simulink model "problem8"  (R2020b)
settings: Solver=VariableStepAuto  StartTime=0.0  StopTime=20  RelTol=1e-3
libraries: simulink x1
settings Model: EnablePacing=on  Creator=INDRAJIT MARATHE  LastModifiedBy=Acer

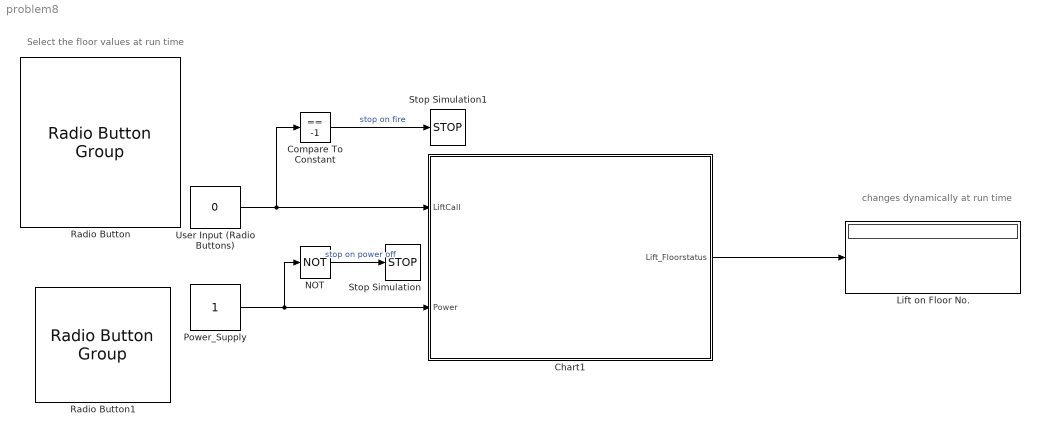
== system problem8 ==
  note: changes dynamically at run time
  note: Select the floor values at run time
  Chart1 : Stateflow chart  TreatAsAtomicUnit=on
  Compare To Constant : simulink/Logic and Bit Operations/Compare To Constant  relop===  const=-1  OutDataTypeStr=boolean
  Lift on Floor No. : Display
  NOT : Logic  Operator=NOT  IconShape=distinctive  AllPortsSameDT=off  OutDataTypeStr=boolean
  Power_Supply : Constant
  Radio Button : RadioButtonGroup  SelectedLabel=Ground Floor  ButtonGroupName=Lift Dashboard
      settings: Values={{'1', '2', '3', '4', '5', 'Ground Floor', 'Fire'}, [1 2 3 4 5 0 -1]}
  Radio Button1 : RadioButtonGroup  SelectedLabel=On  ButtonGroupName=Power Supply
      settings: Values={{'On', 'Off'}, [1 0]}
  Stop Simulation : Stop
  Stop Simulation1 : Stop
  User Input (Radio Buttons) : Constant  Value=0
  wires:
  Power_Supply/1 -> NOT/1, Chart1/2(Power)
  Chart1/1(Lift_Floorstatus) -> Lift on Floor No./1
  User Input (Radio Buttons)/1 -> Compare To Constant/1, Chart1/1(LiftCall)
  NOT/1 -> Stop Simulation/1  "stop on power off"
  Compare To Constant/1 -> Stop Simulation1/1  "stop on fire"

== stateflow chart problem8/Chart1 ==
  state PowerControl [parallel]
    settings: executionOrder=1
    state Idle
      Lift_Floorstatus=0;
    state Active
    (default) -> Idle : {Lift_Floorstatus=1;}
    Idle -> Active : [Power ==1]
    Active -> Idle : [Power==0]
  state Lift_Status [parallel]
    settings: executionOrder=2
    state Up
      du:Lift_Floorstatus=Lift_Floorstatus+1;
    state Start
    state Down
      du:Lift_Floorstatus=Lift_Floorstatus-1;
    state Wait
    Down -> (junction 43) [order 2]
    (default) -> Start
    Up -> (junction 43) [order 2]
    Start -> Up [order 2] : [LiftCall>Lift_Floorstatus && Lift_Floorstatus<5]
    Start -> Down [order 1] : [LiftCall<Lift_Floorstatus && Lift_Floorstatus>0]
    Down -> Wait [order 1] : [Lift_Floorstatus==LiftCall]
    Wait -> Start : after(1,sec)
    Up -> Wait [order 1] : [Lift_Floorstatus==LiftCall]
  data: Lift_Floorstatus output; LiftCall input; Power input
